simulink model "tril_solar"  (R2022a)
settings: Solver=VariableStepAuto  StartTime=0.0  StopTime=1  RelTol=1e-3
libraries: spsVoltageMeasurementLib x3, spsSeriesRLCBranchLib x2, spsCurrentMeasurementLib x2, spsPVArrayLib x1, spspowerguiLib x1
settings Model: Creator=nikke  LastModifiedBy=nikke

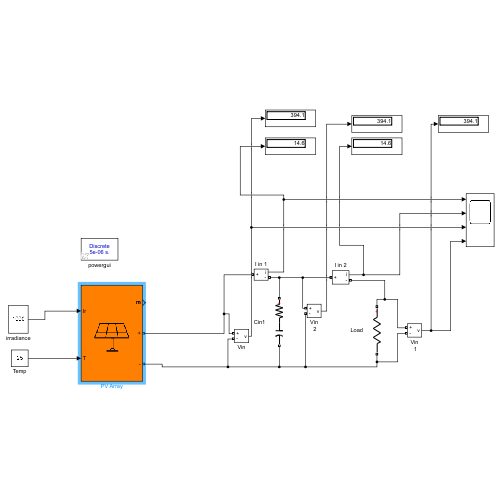
[thumbnail: Simulink's stored preview of the top-level diagram]
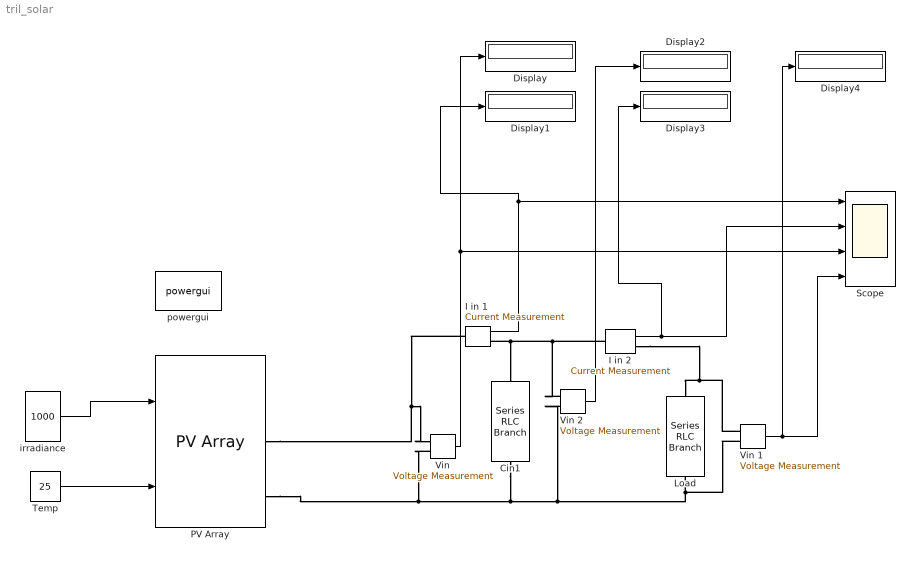
== system tril_solar ==
  Cin1 : spsSeriesRLCBranchLib/Series RLC Branch  LConnTagsString=__new0  RConnTagsString=__new0  BranchType=RC  Resistance=1e-4  Inductance=1e-3  SetiL0=off  InitialCurrent=0  Capacitance=100e-6  Setx0=off  InitialVoltage=0  Measurements=None
  Display{,1..4} (5 alike) : Display
  I in 1 : spsCurrentMeasurementLib/Current Measurement  PhasorSimulation=off  OutputType=Complex  PSBequivalent=0
  I in 2 : spsCurrentMeasurementLib/Current Measurement  PhasorSimulation=off  OutputType=Complex  PSBequivalent=0
  Load : spsSeriesRLCBranchLib/Series RLC Branch  LConnTagsString=__new0  RConnTagsString=__new0  BranchType=R  Resistance=27  Inductance=1e-3  SetiL0=off  InitialCurrent=0  Capacitance=100e-6  Setx0=off  InitialVoltage=0  Measurements=None
  PV Array : spsPVArrayLib/PV Array  Npar=4  Nser=11  PlotType=array @ 25 deg.C & specified irradiances  S_vec=[ 1000]  Temp_C_vec="[ 45 25  ]"  ModuleName=Trina Solar TSM-250PA05.08  PlotWhenSelected=off  Pm=249.86  Ncell=60  Voc=37.6  Isc=8.55  Vm=31  Im=8.06  beta_Voc_pc=-0.35  alpha_Isc_pc=0.06  beta_Voc=-0.1316  alpha_Isc=0.00513  IL=8.5795  I0=2.0381e-10  nI=0.99766  Rsh=301.8149  Rs=0.247  RobustModel=off  RobustCellTemperature=313.3991  BAL=on  Tc=1e-6  Tfilter=1e-5
  Scope : Scope  NumInputPorts=4
  "Temp " : Constant  Value=25
  "Vin " : spsVoltageMeasurementLib/Voltage Measurement  PhasorSimulation=off  OutputType=Complex  PSBequivalent=0
  Vin 1 : spsVoltageMeasurementLib/Voltage Measurement  PhasorSimulation=off  OutputType=Complex  PSBequivalent=0
  Vin 2 : spsVoltageMeasurementLib/Voltage Measurement  PhasorSimulation=off  OutputType=Complex  PSBequivalent=0
  irradiance : Constant  Value=1000  SampleTime=1
  powergui : spspowerguiLib/powergui  Priority=1  SimulationMode=Discrete  SampleTime=5e-6  frequency=60  Iterations=50  frequencyindice=0  Pbase=100e6  ErrMax=1e-4  UnitsV=kV  UnitsW=MW  buscounter=0  FunctionMessages=off  echomessages=off  EnableUseOfTLC=off  CurrentSourceSwitches=off  DisableSnubberDevices=off  DisableRonSwitches=off  DisableVfSwitches=off  DisplayEquations=off  AutomaticDiscreteSolvers=off  SolverType=Tustin/Backward Euler (TBE)  Interpol=off  ExternalGateDelay=off  methode=off  Ts=10  x0status=blocks  SPID=off  SwTol=0  HookPort=off  NonlinearTolerance=1e-4  nMaxIteration=100  ContinueOnMaxIteration=off  RestoreLinks=warning  ResistiveCurrentMeasurement=off  Frange=[0:2:500]  Ylog=off  Xlog=on  ShowGrid=off  save=off  variable=ZData  structure=0  ZoomFFT=off  StartTime=0.0  cycles=1  DisplayStyle=1  fundamental=60  FreqAxis=off  MaxFrequency=1000  frequencyindicesteady=1  RmsSteady=1  display=off
  wires:
  "Temp "/1 -> PV Array/2
  irradiance/1 -> PV Array/1
  Vin 2/1 -> Display2/1
  "Vin "/1 -> Display/1, Scope/3
  Vin 1/1 -> Display4/1, Scope/4
  I in 2/1 -> Display3/1, Scope/2
  I in 1/1 -> Scope/1, Display1/1
  connections:
  Load/LConn1 -- Vin 1/LConn1 -- I in 2/RConn1
  I in 2/LConn1 -- Cin1/LConn1 -- I in 1/RConn1 -- Vin 2/LConn1
  Load/RConn1 -- Vin 1/LConn2 -- Vin 2/LConn2 -- Cin1/RConn1 -- PV Array/RConn2 -- "Vin "/LConn2
  "Vin "/LConn1 -- PV Array/RConn1 -- I in 1/LConn1
